simulink model "Fuchs_FDFR_simulink_nonlinear"  (R2024a)
settings: Solver=ode4  StartTime=0.0  StopTime=300  FixedStep=0.02  RelTol=1e-3
libraries: vrlib x1
(part 3 of 3)

== system Fuchs_FDFR_simulink_nonlinear/Strecke/get_rho_of_alt1 ==
  IN_env : Inport
  IN_alt_m : Inport  Port=2
  Bus Selector : BusSelector  OutputSignals=rho_0,y_H,T_0,g,R
  MATLAB Function : MATLAB Function  TreatAsAtomicUnit=on
  rho : Outport
  wires:
  IN_alt_m/1 -> MATLAB Function/6(altitude_m)
  IN_env/1 -> Bus Selector/1
  Bus Selector/1 -> MATLAB Function/1(rho_0)  "<rho_0>"
  MATLAB Function/1(rho) -> rho/1
  Bus Selector/2 -> MATLAB Function/2(y_H)  "<y_H>"
  Bus Selector/3 -> MATLAB Function/3(T_0)  "<T_0>"
  Bus Selector/4 -> MATLAB Function/4(g)  "<g>"
  Bus Selector/5 -> MATLAB Function/5(R)  "<R>"

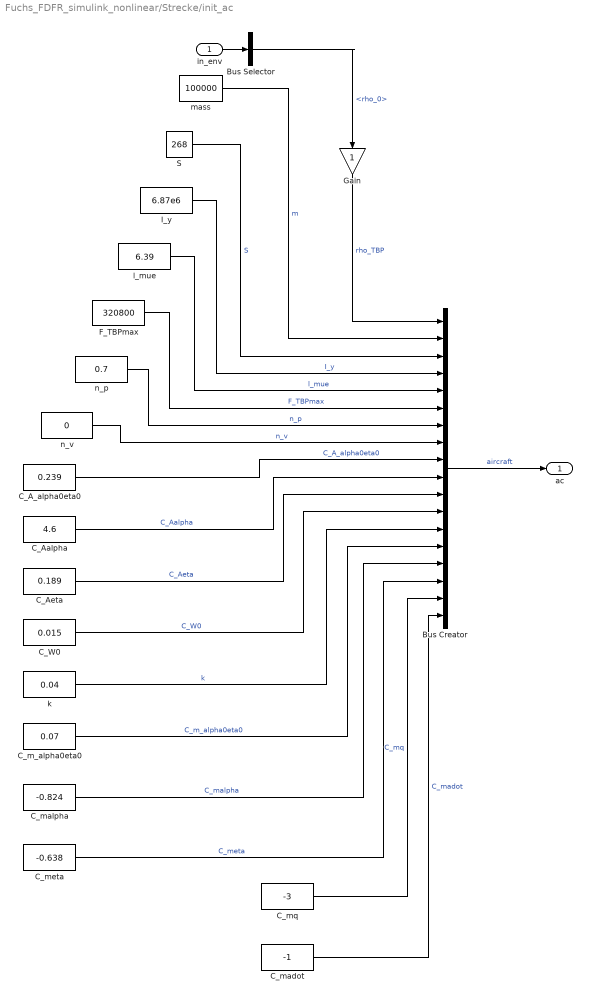
== system Fuchs_FDFR_simulink_nonlinear/Strecke/init_ac ==
  in_env : Inport
  Bus Creator : BusCreator  Inputs=18
  Bus Selector : BusSelector  OutputSignals=rho_0
  C_A_alpha0eta0 : Constant  Value=0.239
  C_Aalpha : Constant  Value=4.6
  C_Aeta : Constant  Value=0.189
  C_W0 : Constant  Value=0.015
  C_m_alpha0eta0 : Constant  Value=0.07
  C_madot : Constant  Value=-1
  C_malpha : Constant  Value=-0.824
  C_meta : Constant  Value=-0.638
  C_mq : Constant  Value=-3
  F_TBPmax : Constant  Value=320800
  Gain : Gain
  I_y : Constant  Value=6.87e6
  S : Constant  Value=268
  k : Constant  Value=0.04
  l_mue : Constant  Value=6.39
  mass : Constant  Value=100000
  n_p : Constant  Value=0.7
  n_v : Constant  Value=0
  ac : Outport
  wires:
  in_env/1 -> Bus Selector/1
  Bus Selector/1 -> Gain/1  "<rho_0>"
  Bus Creator/1 -> ac/1  "aircraft"
  mass/1 -> Bus Creator/2  "m"
  S/1 -> Bus Creator/3  "S"
  I_y/1 -> Bus Creator/4  "I_y"
  l_mue/1 -> Bus Creator/5  "l_mue"
  F_TBPmax/1 -> Bus Creator/6  "F_TBPmax"
  n_p/1 -> Bus Creator/7  "n_p"
  n_v/1 -> Bus Creator/8  "n_v"
  C_A_alpha0eta0/1 -> Bus Creator/9  "C_A_alpha0eta0"
  C_Aalpha/1 -> Bus Creator/10  "C_Aalpha"
  C_Aeta/1 -> Bus Creator/11  "C_Aeta"
  C_W0/1 -> Bus Creator/12  "C_W0"
  k/1 -> Bus Creator/13  "k"
  C_m_alpha0eta0/1 -> Bus Creator/14  "C_m_alpha0eta0"
  C_malpha/1 -> Bus Creator/15  "C_malpha"
  C_meta/1 -> Bus Creator/16  "C_meta"
  C_mq/1 -> Bus Creator/17  "C_mq"
  C_madot/1 -> Bus Creator/18  "C_madot"
  Gain/1 -> Bus Creator/1  "rho_TBP"

== system Fuchs_FDFR_simulink_nonlinear/Strecke/init_env ==
  Bus Creator : BusCreator  Inputs=5
  R : Constant  Value=287.058
  T_0 : Constant  Value=288.15
  g : Constant  Value=9.81
  rho_0 : Constant  Value=1.225
  y_H : Constant  Value=-0.0065
  env : Outport
  wires:
  Bus Creator/1 -> env/1  "enviroment"
  g/1 -> Bus Creator/1  "g"
  rho_0/1 -> Bus Creator/2  "rho_0"
  R/1 -> Bus Creator/3  "R"
  T_0/1 -> Bus Creator/4  "T_0"
  y_H/1 -> Bus Creator/5  "y_H"

== system Fuchs_FDFR_simulink_nonlinear/Strecke/Beiwerte/Auftriebsbeiwert ==
  IN_steuer : Inport
  IN_zg : Inport  Port=2
  IN_ac : Inport  Port=3
  Bus Selector : BusSelector  OutputSignals=eta
  Bus Selector1 : BusSelector  OutputSignals=alpha
  Bus Selector2 : BusSelector  OutputSignals=C_A_alpha0eta0,C_Aalpha,C_Aeta
  MATLAB Function : MATLAB Function  TreatAsAtomicUnit=on
  OUT_C_A : Outport
  wires:
  IN_steuer/1 -> Bus Selector/1
  Bus Selector/1 -> MATLAB Function/5(eta)  "<eta>"
  IN_zg/1 -> Bus Selector1/1
  Bus Selector1/1 -> MATLAB Function/4(alpha)  "<alpha>"
  IN_ac/1 -> Bus Selector2/1
  MATLAB Function/1(c_A) -> OUT_C_A/1
  Bus Selector2/3 -> MATLAB Function/3(C_Aeta)  "<C_Aeta>"
  Bus Selector2/2 -> MATLAB Function/2(C_Aalpha)  "<C_Aalpha>"
  Bus Selector2/1 -> MATLAB Function/1(C_A_alpha0eta0)  "<C_A_alpha0eta0>"

== system Fuchs_FDFR_simulink_nonlinear/Strecke/Beiwerte/Nickmomentbeiwert ==
  IN_steuer : Inport
  IN_zg : Inport  Port=2
  IN_ac : Inport  Port=3
  IN_zustandsgroessen_dot : Inport  Port=4
  Bus Selector : BusSelector  OutputSignals=C_m_alpha0eta0,C_malpha,C_meta,C_mq,C_madot,l_mue
  Bus Selector1 : BusSelector  OutputSignals=alpha,q,V
  Bus Selector2 : BusSelector  OutputSignals=alpha_dot
  Bus Selector3 : BusSelector  OutputSignals=eta
  MATLAB Function : MATLAB Function  TreatAsAtomicUnit=on
  OUT_C_m : Outport
  wires:
  MATLAB Function/1(C_m) -> OUT_C_m/1
  IN_ac/1 -> Bus Selector/1
  Bus Selector/1 -> MATLAB Function/1(C_m_alpha0eta0)  "<C_m_alpha0eta0>"
  Bus Selector/2 -> MATLAB Function/2(C_malpha)  "<C_malpha>"
  Bus Selector/3 -> MATLAB Function/3(C_meta)  "<C_meta>"
  Bus Selector/4 -> MATLAB Function/4(C_mq)  "<C_mq>"
  Bus Selector/5 -> MATLAB Function/5(C_malphadot)  "<C_madot>"
  Bus Selector/6 -> MATLAB Function/6(l_mue)  "<l_mue>"
  IN_zg/1 -> Bus Selector1/1
  Bus Selector1/1 -> MATLAB Function/7(alpha)  "<alpha>"
  Bus Selector1/2 -> MATLAB Function/8(q)  "<q>"
  Bus Selector1/3 -> MATLAB Function/9(V)  "<V>"
  IN_zustandsgroessen_dot/1 -> Bus Selector2/1
  Bus Selector2/1 -> MATLAB Function/10(alpha_dot)  "<alpha_dot>"
  IN_steuer/1 -> Bus Selector3/1
  Bus Selector3/1 -> MATLAB Function/11(eta)  "<eta>"

== system Fuchs_FDFR_simulink_nonlinear/Strecke/Beiwerte/Widerstandsbeiwert ==
  IN_C_A : Inport
  IN_ac : Inport  Port=2
  Bus Selector : BusSelector  OutputSignals=C_W0,k
  MATLAB Function : MATLAB Function  TreatAsAtomicUnit=on
  OUT_C_W : Outport
  wires:
  MATLAB Function/1(C_W) -> OUT_C_W/1
  IN_C_A/1 -> MATLAB Function/1(C_A)
  IN_ac/1 -> Bus Selector/1
  Bus Selector/1 -> MATLAB Function/2(C_W0)  "<C_W0>"
  Bus Selector/2 -> MATLAB Function/3(k)  "<k>"

== system Fuchs_FDFR_simulink_nonlinear/Strecke/DGL/H_dot ==
  IN_zustandsgroessen : Inport
  Bus Selector3 : BusSelector  OutputSignals=y,V
  H_dot : MATLAB Function  TreatAsAtomicUnit=on
  OUT_H_dot : Outport
  wires:
  Bus Selector3/1 -> H_dot/1(y)  "<y>"
  Bus Selector3/2 -> H_dot/2(V)  "<V>"
  IN_zustandsgroessen/1 -> Bus Selector3/1
  H_dot/1(H_dot) -> OUT_H_dot/1

== system Fuchs_FDFR_simulink_nonlinear/Strecke/DGL/R_dotz ==
  IN_zustandsgroessen : Inport
  Bus Selector3 : BusSelector  OutputSignals=y,V
  R_dot : MATLAB Function  TreatAsAtomicUnit=on
  OUT_R_dot : Outport
  wires:
  Bus Selector3/1 -> R_dot/1(y)  "<y>"
  Bus Selector3/2 -> R_dot/2(V)  "<V>"
  IN_zustandsgroessen/1 -> Bus Selector3/1
  R_dot/1(R_dot) -> OUT_R_dot/1

== system Fuchs_FDFR_simulink_nonlinear/Strecke/DGL/alpha_dot ==
  IN_y_dot : Inport
  IN_zustandsgroessen : Inport  Port=2
  Bus Selector3 : BusSelector  OutputSignals=q
  alpha_dot : MATLAB Function  TreatAsAtomicUnit=on
  OUT_alpha_dot : Outport
  wires:
  IN_zustandsgroessen/1 -> Bus Selector3/1
  alpha_dot/1(alpha_dot) -> OUT_alpha_dot/1
  IN_y_dot/1 -> alpha_dot/2(y_dot)
  Bus Selector3/1 -> alpha_dot/1(q)  "<q>"

== system Fuchs_FDFR_simulink_nonlinear/Strecke/DGL/q_dot ==
  IN_ac : Inport
  IN_kraefte_momente : Inport  Port=2
  Bus Selector1 : BusSelector  OutputSignals=I_y
  Bus Selector2 : BusSelector  OutputSignals=M
  q_dot : MATLAB Function  TreatAsAtomicUnit=on
  OUT_q_dot : Outport
  wires:
  IN_kraefte_momente/1 -> Bus Selector2/1
  IN_ac/1 -> Bus Selector1/1
  q_dot/1(q_dot) -> OUT_q_dot/1
  Bus Selector2/1 -> q_dot/1(M)  "<M>"
  Bus Selector1/1 -> q_dot/2(I_y)  "<I_y>"

== system Fuchs_FDFR_simulink_nonlinear/Strecke/DGL/v_dot ==
  IN_env : Inport
  IN_ac : Inport  Port=2
  IN_kraefte_momente : Inport  Port=3
  IN_zustandsgroessen : Inport  Port=4
  Bus Selector : BusSelector  OutputSignals=g
  Bus Selector1 : BusSelector  OutputSignals=m
  Bus Selector2 : BusSelector  OutputSignals=W,F
  Bus Selector3 : BusSelector  OutputSignals=y,alpha
  v_dot : MATLAB Function  TreatAsAtomicUnit=on
  OUT_v_dot : Outport
  wires:
  Bus Selector3/1 -> v_dot/5(y)  "<y>"
  Bus Selector3/2 -> v_dot/6(alpha)  "<alpha>"
  Bus Selector/1 -> v_dot/2(g)  "<g>"
  Bus Selector2/2 -> v_dot/4(F)  "<F>"
  Bus Selector1/1 -> v_dot/1(m)  "<m>"
  IN_env/1 -> Bus Selector/1
  IN_kraefte_momente/1 -> Bus Selector2/1
  Bus Selector2/1 -> v_dot/3(W)  "<W>"
  IN_zustandsgroessen/1 -> Bus Selector3/1
  IN_ac/1 -> Bus Selector1/1
  v_dot/1(v_dot) -> OUT_v_dot/1

== system Fuchs_FDFR_simulink_nonlinear/Strecke/DGL/y_dot ==
  IN_env : Inport
  IN_ac : Inport  Port=2
  IN_kraefte_momente : Inport  Port=3
  IN_zustandsgroessen : Inport  Port=4
  Bus Selector : BusSelector  OutputSignals=g
  Bus Selector1 : BusSelector  OutputSignals=m
  Bus Selector2 : BusSelector  OutputSignals=A,F
  Bus Selector3 : BusSelector  OutputSignals=y,alpha,V
  y_dot : MATLAB Function  TreatAsAtomicUnit=on
  OUT_y_dot : Outport
  wires:
  Bus Selector/1 -> y_dot/2(g)  "<g>"
  Bus Selector2/2 -> y_dot/4(F)  "<F>"
  Bus Selector1/1 -> y_dot/1(m)  "<m>"
  IN_env/1 -> Bus Selector/1
  IN_kraefte_momente/1 -> Bus Selector2/1
  Bus Selector2/1 -> y_dot/3(A)  "<A>"
  IN_zustandsgroessen/1 -> Bus Selector3/1
  IN_ac/1 -> Bus Selector1/1
  y_dot/1(y_dot) -> OUT_y_dot/1  "y_dot"
  Bus Selector3/2 -> y_dot/6(alpha)  "<alpha>"
  Bus Selector3/1 -> y_dot/5(y)  "<y>"
  Bus Selector3/3 -> y_dot/7(V)  "<V>"

== system Fuchs_FDFR_simulink_nonlinear/Strecke/Kraefte_Momente/Auftrieb ==
  IN_bw : Inport
  IN_zg : Inport  Port=2
  IN_ac : Inport  Port=3
  IN_rho : Inport  Port=4
  A : MATLAB Function  TreatAsAtomicUnit=on
  Bus Selector : BusSelector  OutputSignals=C_A
  Bus Selector1 : BusSelector  OutputSignals=S
  Bus Selector2 : BusSelector  OutputSignals=V
  OUT_A : Outport
  wires:
  IN_bw/1 -> Bus Selector/1
  IN_ac/1 -> Bus Selector1/1
  Bus Selector1/1 -> A/2(S)  "<S>"
  IN_zg/1 -> Bus Selector2/1
  Bus Selector2/1 -> A/3(V)  "<V>"
  IN_rho/1 -> A/4(rho)  "rho"
  A/1(A) -> OUT_A/1
  Bus Selector/1 -> A/1(C_A)  "<C_A>"

== system Fuchs_FDFR_simulink_nonlinear/Strecke/Kraefte_Momente/Nickmoment ==
  IN_bw : Inport
  IN_zg : Inport  Port=2
  IN_ac : Inport  Port=3
  IN_rho : Inport  Port=4
  Bus Selector : BusSelector  OutputSignals=C_m
  Bus Selector1 : BusSelector  OutputSignals=S,l_mue
  Bus Selector2 : BusSelector  OutputSignals=V
  M : MATLAB Function  TreatAsAtomicUnit=on
  OUT_M : Outport
  wires:
  IN_bw/1 -> Bus Selector/1
  Bus Selector/1 -> M/1(C_m)  "<C_m>"
  IN_ac/1 -> Bus Selector1/1
  Bus Selector1/1 -> M/2(S)  "<S>"
  IN_zg/1 -> Bus Selector2/1
  Bus Selector2/1 -> M/4(V)  "<V>"
  IN_rho/1 -> M/5(rho)  "rho"
  M/1(M) -> OUT_M/1
  Bus Selector1/2 -> M/3(l_mue)  "<l_mue>"

== system Fuchs_FDFR_simulink_nonlinear/Strecke/Kraefte_Momente/Schub ==
  IN_steuer : Inport
  IN_ac : Inport  Port=2
  IN_rho : Inport  Port=3
  Bus Selector1 : BusSelector  OutputSignals=rho_TBP,F_TBPmax,n_p
  Bus Selector2 : BusSelector  OutputSignals=delta
  F : MATLAB Function  TreatAsAtomicUnit=on
  OUT_F : Outport
  wires:
  IN_ac/1 -> Bus Selector1/1
  Bus Selector1/1 -> F/1(rho_TBP)  "<rho_TBP>"
  IN_steuer/1 -> Bus Selector2/1
  Bus Selector2/1 -> F/4(delta)  "<delta>"
  IN_rho/1 -> F/5(rho)  "rho"
  F/1(F) -> OUT_F/1
  Bus Selector1/2 -> F/2(F_TBPmax)  "<F_TBPmax>"
  Bus Selector1/3 -> F/3(n_p)  "<n_p>"

== system Fuchs_FDFR_simulink_nonlinear/Strecke/Kraefte_Momente/Widerstand ==
  IN_bw : Inport
  IN_zg : Inport  Port=2
  IN_ac : Inport  Port=3
  IN_rho : Inport  Port=4
  Bus Selector : BusSelector  OutputSignals=C_W
  Bus Selector1 : BusSelector  OutputSignals=S
  Bus Selector2 : BusSelector  OutputSignals=V
  W : MATLAB Function  TreatAsAtomicUnit=on
  OUT_W : Outport
  wires:
  IN_bw/1 -> Bus Selector/1
  Bus Selector/1 -> W/1(C_W)  "<C_W>"
  IN_ac/1 -> Bus Selector1/1
  Bus Selector1/1 -> W/2(S)  "<S>"
  IN_zg/1 -> Bus Selector2/1
  Bus Selector2/1 -> W/3(V)  "<V>"
  IN_rho/1 -> W/4(rho)  "rho"
  W/1(W) -> OUT_W/1

== matlab function Fuchs_FDFR_simulink_nonlinear/Strecke/Kraefte_Momente/Nickmoment/M ==
  data: C_m input; S input; l_mue input; V input; M output; rho input
function M = fcn(C_m, S, l_mue, V, rho)

M = C_m*(rho/2)*power(V,2)*S*l_mue;

== matlab function Fuchs_FDFR_simulink_nonlinear/Strecke/Kraefte_Momente/Schub/F ==
  data: rho_TBP input; F_TBPmax input; n_p input; delta input; F output; rho input
function F = fcn(rho_TBP, F_TBPmax, n_p, delta, rho)

F = delta*F_TBPmax*power((rho/rho_TBP), n_p);

== matlab function Fuchs_FDFR_simulink_nonlinear/Strecke/Beiwerte/Auftriebsbeiwert/MATLAB Function ==
  data: C_A_alpha0eta0 input; c_A output; C_Aalpha input; C_Aeta input; alpha input; eta input
function c_A = fcn(C_A_alpha0eta0, C_Aalpha, C_Aeta, alpha, eta)

c_A = C_A_alpha0eta0 + C_Aalpha*alpha + C_Aeta*eta;

== matlab function Fuchs_FDFR_simulink_nonlinear/Strecke/Beiwerte/Widerstandsbeiwert/MATLAB Function ==
  data: C_A input; C_W output; C_W0 input; k input
function C_W = fcn(C_A, C_W0, k)

C_W = C_W0 + k*power(C_A,2);

== matlab function Fuchs_FDFR_simulink_nonlinear/Strecke/Beiwerte/Nickmomentbeiwert/MATLAB Function ==
  data: C_m_alpha0eta0 input; C_m output; C_malpha input; C_meta input; C_mq input; C_malphadot input; l_mue input; alpha input; q input; V input; alpha_dot input; eta input
function C_m = fcn(C_m_alpha0eta0, C_malpha, C_meta, C_mq, C_malphadot, l_mue, alpha, q, V, alpha_dot, eta)

C_m = C_m_alpha0eta0 + C_malpha*alpha + C_meta*eta + (C_mq*q + C_malphadot*alpha_dot)*(l_mue/V);

== matlab function Fuchs_FDFR_simulink_nonlinear/Strecke/get_rho_of_alt1/MATLAB Function ==
  data: rho_0 input; rho output; y_H input; T_0 input; g input; R input; altitude_m input
function rho = fcn(rho_0, y_H, T_0, g, R, altitude_m)
    rho = rho_0 * power((1+ (y_H/T_0)*altitude_m),(-(g/(R*y_H))-1));

== matlab function Fuchs_FDFR_simulink_nonlinear/Strecke/DGL/v_dot/v_dot ==
  data: m input; g input; W input; v_dot output; F input; y input; alpha input
function v_dot= fcn(m, g, W, F, y, alpha)

v_dot = -(W/m)-g*sin(y)+(F/m)*cos(alpha);

== matlab function Fuchs_FDFR_simulink_nonlinear/Strecke/DGL/y_dot/y_dot ==
  data: m input; g input; A input; y_dot output; F input; y input; alpha input; V input
function y_dot= fcn(m, g, A, F, y, alpha, V)

y_dot = (A/(m*V))-(g/V)*cos(y)+(F/(m*V))*sin(alpha);

== matlab function Fuchs_FDFR_simulink_nonlinear/Strecke/DGL/q_dot/q_dot ==
  data: M input; I_y input; q_dot output
function q_dot= fcn(M, I_y)

q_dot = M/I_y;

== matlab function Fuchs_FDFR_simulink_nonlinear/Strecke/DGL/alpha_dot/alpha_dot ==
  data: q input; y_dot input; alpha_dot output
function alpha_dot= fcn(q, y_dot)

alpha_dot = q - y_dot;

== matlab function Fuchs_FDFR_simulink_nonlinear/Strecke/DGL/H_dot/H_dot ==
  data: y input; V input; H_dot output
function H_dot= fcn(y, V)

H_dot = V*sin(y);

== matlab function Fuchs_FDFR_simulink_nonlinear/Strecke/DGL/R_dotz/R_dot ==
  data: y input; V input; R_dot output
function R_dot= fcn(y, V)

R_dot = V*cos(y);

== matlab function Fuchs_FDFR_simulink_nonlinear/Strecke/Kraefte_Momente/Auftrieb/A ==
  data: C_A input; S input; V input; A output; rho input
function A = fcn(C_A, S, V, rho)

A = C_A*(rho/2)*power(V,2)*S;

== matlab function Fuchs_FDFR_simulink_nonlinear/Strecke/Kraefte_Momente/Widerstand/W ==
  data: C_W input; S input; V input; W output; rho input
function W = fcn(C_W, S, V, rho)

W = C_W*(rho/2)*power(V,2)*S;
